simulink model "BRLab"  (R2022b)
settings: Solver=FixedStepDiscrete  StartTime=0.0  StopTime=60  FixedStep=0.01  RelTol=1e-3
undefined symbols (not defined in the file or in its folder): controller, DiscIntNeverNeededParam, drv, filt, gbox, sens, Ts, wheel, yaw
settings Model: Creator=Alessandro  LastModifiedBy=michael
settings SolverCC: AlgebraicLoopSolver=TrustRegion
settings ModelReferenceCC: EnableRefExpFcnMdlSchedulingChecks=on
settings RTWCC: DLArmComputeVersion=19.05

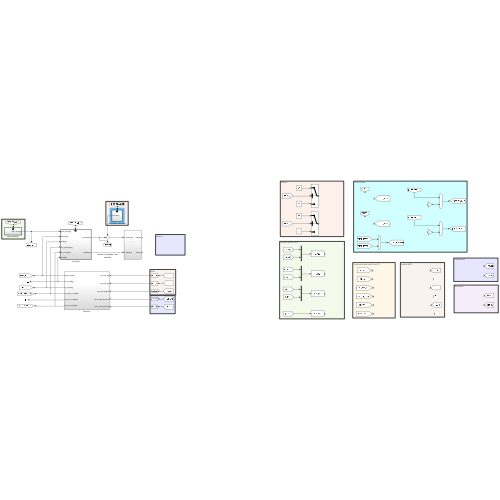
[thumbnail: Simulink's stored preview of the top-level diagram]
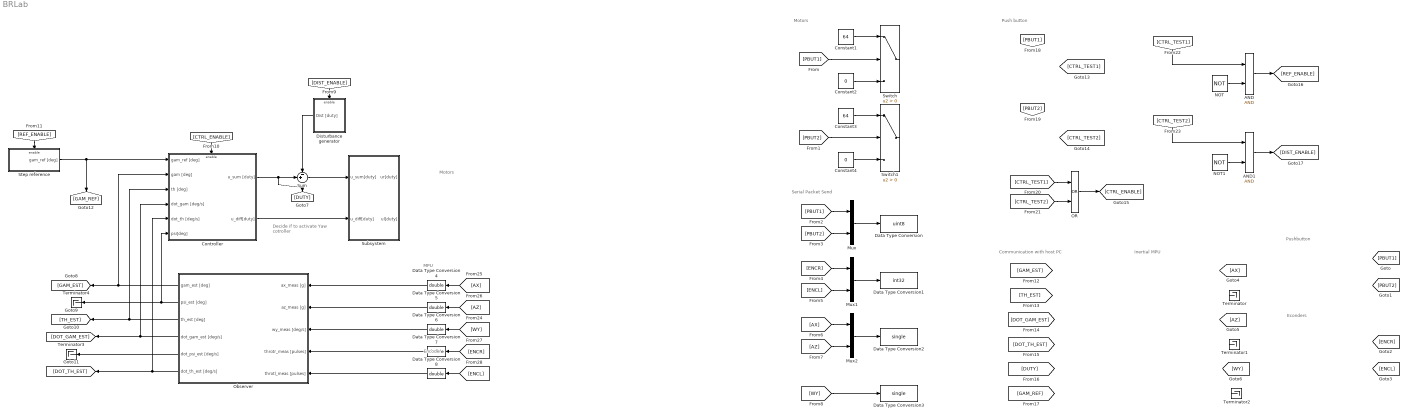
== system BRLab ==
  note: Encoder
  note: MPU
  note: Push button
  note: Communication with host PC
  note: Motors
  note: Decide if to activate Yaw cotroller
  note: Serial Packet Send
  note: Econders
  note: Pushbutton
  note: Motors
  note: Inertial MPU
  AND : Logic  IconShape=distinctive  AllPortsSameDT=off  OutDataTypeStr=boolean
  AND1 : Logic  IconShape=distinctive  AllPortsSameDT=off  OutDataTypeStr=boolean
  Constant1 : Constant  Value=64
  Constant2 : Constant  Value=0
  Constant3 : Constant  Value=64
  Constant4 : Constant  Value=0
  Controller : Subsystem
  Data Type Conversion : DataTypeConversion  OutDataTypeStr=uint8  SaturateOnIntegerOverflow=off  RndMeth=Floor
  Data Type Conversion1 : DataTypeConversion  OutDataTypeStr=int32  SaturateOnIntegerOverflow=off  RndMeth=Floor
  Data Type Conversion2 : DataTypeConversion  OutDataTypeStr=single  SaturateOnIntegerOverflow=off  RndMeth=Floor
  Data Type Conversion3 : DataTypeConversion  OutDataTypeStr=single  SaturateOnIntegerOverflow=off  RndMeth=Floor
  Data Type Conversion{4..8} (5 alike) : DataTypeConversion  OutDataTypeStr=double  SaturateOnIntegerOverflow=off  RndMeth=Floor
  Disturbance generator : Subsystem
  Mux : Mux  Inputs=2
  Mux1 : Mux  Inputs=2
  Mux2 : Mux  Inputs=2
  NOT : Logic  Operator=NOT  IconShape=distinctive  AllPortsSameDT=off  OutDataTypeStr=boolean
  NOT1 : Logic  Operator=NOT  IconShape=distinctive  AllPortsSameDT=off  OutDataTypeStr=boolean
  OR : Logic  Operator=OR  IconShape=distinctive  AllPortsSameDT=off  OutDataTypeStr=boolean
  Observer : Subsystem
  "Step reference " : Subsystem
  Subsystem : Subsystem
  Sum : Sum  Inputs=-+|
  Switch : Switch  Criteria=u2 > Threshold  SaturateOnIntegerOverflow=off  InputSameDT=off
  Switch1 : Switch  Criteria=u2 > Threshold  SaturateOnIntegerOverflow=off  InputSameDT=off
  Terminator{,1..4} (5 alike) : Terminator
  wires:
  Controller/1(u_sum [duty]) -> [DUTY], Sum/2
  Observer/1(gam_est [deg]) -> Controller/2(gam [deg]), [GAM_EST]
  Sum/1 -> Subsystem/1(u_sum[duty])
  Observer/3(th_est [deg]) -> Controller/3(th [deg]), [TH_EST]
  Observer/6(dot_th_est [deg/s]) -> Controller/5(dot_th [deg/s]), [DOT_TH_EST]
  Observer/4(dot_gam_est [deg/s]) -> Controller/4(dot_gam [deg/s]), [DOT_GAM_EST]
  Observer/2(psi_est [deg]) -> Controller/6(psi[deg]), Terminator4/1
  "Step reference "/1(gam_ref [deg]) -> [GAM_REF], Controller/1(gam_ref [deg])
  Controller/2(u_diff[duty]) -> Subsystem/2(u_diff[duty])
  [PBUT1] -> Mux/1
  [WY] -> Data Type Conversion3/1
  Constant1/1 -> Switch/1
  [PBUT1] -> Switch/2
  Constant3/1 -> Switch1/1
  Mux/1 -> Data Type Conversion/1
  [AX] -> Mux2/1
  [ENCL] -> Mux1/2
  [PBUT2] -> Mux/2
  [ENCR] -> Mux1/1
  Mux1/1 -> Data Type Conversion1/1
  Constant4/1 -> Switch1/3
  [PBUT2] -> Switch1/2
  Constant2/1 -> Switch/3
  Mux2/1 -> Data Type Conversion2/1
  [AZ] -> Mux2/2
  Disturbance generator/1(Dist [duty]) -> Sum/1
  [DIST_ENABLE] -> Disturbance generator/Enable
  [CTRL_ENABLE] -> Controller/Enable
  [REF_ENABLE] -> "Step reference "/Enable
  Observer/5(dot_psi_est [deg/s]) -> Terminator3/1
  [CTRL_TEST1] -> OR/1
  [CTRL_TEST2] -> OR/2
  OR/1 -> [CTRL_ENABLE]
  NOT/1 -> AND/2
  [CTRL_TEST1] -> AND/1
  AND/1 -> [REF_ENABLE]
  AND1/1 -> [DIST_ENABLE]
  NOT1/1 -> AND1/2
  [CTRL_TEST2] -> AND1/1
  Data Type Conversion5/1 -> Observer/2(az_meas [g])
  Data Type Conversion4/1 -> Observer/1(ax_meas [g])
  Data Type Conversion6/1 -> Observer/3(wy_meas [deg/s])
  [WY] -> Data Type Conversion6/1
  [AX] -> Data Type Conversion4/1
  [AZ] -> Data Type Conversion5/1
  Data Type Conversion7/1 -> Observer/4(throtr_meas [pulses])
  [ENCR] -> Data Type Conversion7/1
  [ENCL] -> Data Type Conversion8/1
  Data Type Conversion8/1 -> Observer/5(throtl_meas [pulses])

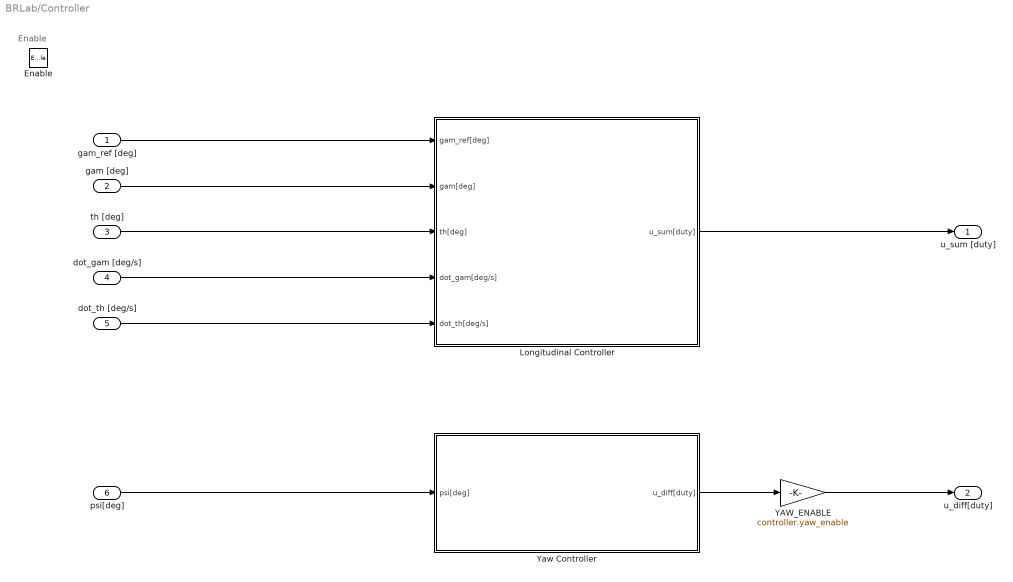
== system BRLab/Controller ==
  note: Enable
  gam_ref [deg] : Inport
  gam [deg] : Inport  Port=2
  th [deg] : Inport  Port=3
  dot_gam [deg/s] : Inport  Port=4
  dot_th [deg/s] : Inport  Port=5
  psi[deg] : Inport  Port=6
  Enable : EnablePort
  Longitudinal Controller : Subsystem
  YAW_ENABLE : Gain  Gain=controller.yaw_enable
  Yaw Controller : Subsystem
  u_sum [duty] : Outport
  u_diff[duty] : Outport  Port=2
  wires:
  psi[deg]/1 -> Yaw Controller/1(psi[deg])
  Yaw Controller/1(u_diff[duty]) -> YAW_ENABLE/1
  gam_ref [deg]/1 -> Longitudinal Controller/1(gam_ref[deg])
  gam [deg]/1 -> Longitudinal Controller/2(gam[deg])
  th [deg]/1 -> Longitudinal Controller/3(th[deg])
  dot_gam [deg/s]/1 -> Longitudinal Controller/4(dot_gam[deg/s])
  dot_th [deg/s]/1 -> Longitudinal Controller/5(dot_th[deg/s])
  Longitudinal Controller/1(u_sum[duty]) -> u_sum [duty]/1
  YAW_ENABLE/1 -> u_diff[duty]/1

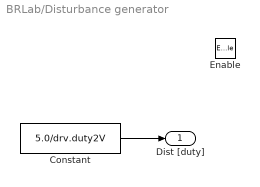
== system BRLab/Disturbance generator ==
  Enable : EnablePort
  Constant : Constant  Value=5.0/drv.duty2V
  Dist [duty] : Outport
  wires:
  Constant/1 -> Dist [duty]/1

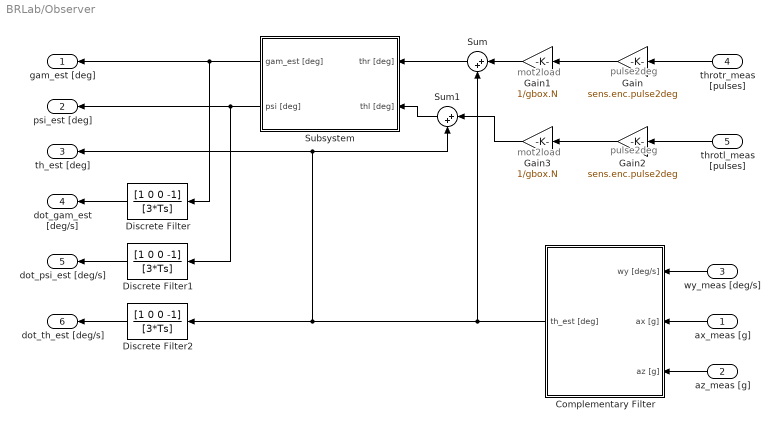
== system BRLab/Observer ==
  note: mot2load
  note: pulse2deg
  note: mot2load
  note: pulse2deg
  ax_meas [g] : Inport
  az_meas [g] : Inport  Port=2
  wy_meas [deg/s] : Inport  Port=3
  throtr_meas [pulses] : Inport  Port=4
  throtl_meas [pulses] : Inport  Port=5
  Complementary Filter : Subsystem
  Discrete Filter : DiscreteFilter  Numerator=[1 0 0 -1]  Denominator=[3*Ts]  SampleTime=Ts
  Discrete Filter1 : DiscreteFilter  Numerator=[1 0 0 -1]  Denominator=[3*Ts]  SampleTime=Ts
  Discrete Filter2 : DiscreteFilter  Numerator=[1 0 0 -1]  Denominator=[3*Ts]  SampleTime=Ts
  Gain : Gain  Gain=sens.enc.pulse2deg
  Gain1 : Gain  Gain=1/gbox.N
  Gain2 : Gain  Gain=sens.enc.pulse2deg
  Gain3 : Gain  Gain=1/gbox.N
  Subsystem : Subsystem
  Sum : Sum  Inputs=|++
  Sum1 : Sum  Inputs=|++
  gam_est [deg] : Outport
  psi_est [deg] : Outport  Port=2
  th_est [deg] : Outport  Port=3
  dot_gam_est [deg/s] : Outport  Port=4
  dot_psi_est [deg/s] : Outport  Port=5
  dot_th_est [deg/s] : Outport  Port=6
  wires:
  Discrete Filter/1 -> dot_gam_est [deg/s]/1
  Gain1/1 -> Sum/1
  Discrete Filter1/1 -> dot_psi_est [deg/s]/1
  Gain/1 -> Gain1/1
  throtr_meas [pulses]/1 -> Gain/1
  wy_meas [deg/s]/1 -> Complementary Filter/1(wy [deg/s])
  Gain2/1 -> Gain3/1
  throtl_meas [pulses]/1 -> Gain2/1
  Gain3/1 -> Sum1/1
  Sum/1 -> Subsystem/1(thr [deg])
  Sum1/1 -> Subsystem/2(thl [deg])
  Complementary Filter/1(th_est [deg]) -> Sum1/2, th_est [deg]/1, Discrete Filter2/1, Sum/2
  Subsystem/2(psi [deg]) -> Discrete Filter1/1, psi_est [deg]/1
  Subsystem/1(gam_est [deg]) -> Discrete Filter/1, gam_est [deg]/1
  Discrete Filter2/1 -> dot_th_est [deg/s]/1
  ax_meas [g]/1 -> Complementary Filter/2(ax [g])
  az_meas [g]/1 -> Complementary Filter/3(az [g])

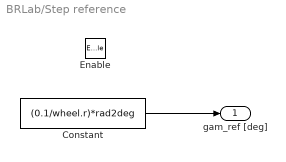
== system BRLab/Step reference  ==
  Enable : EnablePort
  Constant : Constant  Value=(0.1/wheel.r)*rad2deg
  gam_ref [deg] : Outport
  wires:
  Constant/1 -> gam_ref [deg]/1

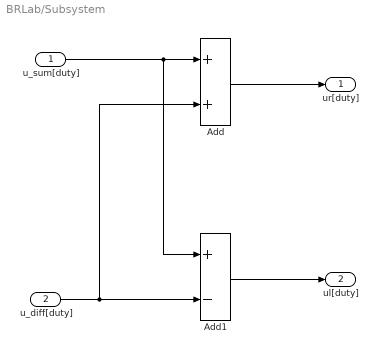
== system BRLab/Subsystem ==
  u_sum[duty] : Inport
  u_diff[duty] : Inport  Port=2
  Add : Sum
  Add1 : Sum  Inputs=+-
  ur[duty] : Outport
  ul[duty] : Outport  Port=2
  wires:
  u_diff[duty]/1 -> Add/2, Add1/2
  Add/1 -> ur[duty]/1
  u_sum[duty]/1 -> Add1/1, Add/1
  Add1/1 -> ul[duty]/1

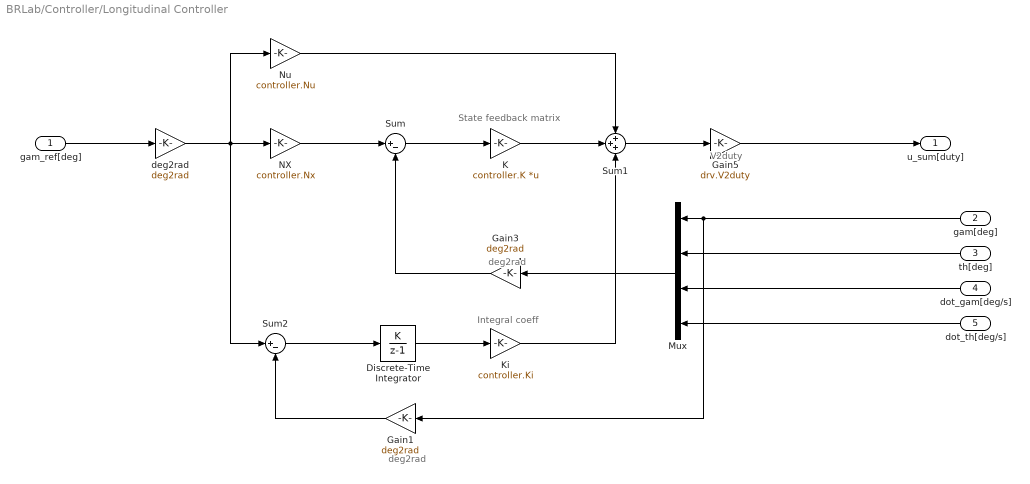
== system BRLab/Controller/Longitudinal Controller ==
  note: State feedback matrix
  note: Integral coeff
  note: V2duty
  note: deg2rad
  note: deg2rad
  gam_ref[deg] : Inport
  gam[deg] : Inport  Port=2
  th[deg] : Inport  Port=3
  dot_gam[deg/s] : Inport  Port=4
  dot_th[deg/s] : Inport  Port=5
  Discrete-Time Integrator : DiscreteIntegrator  IntegratorMethod=Accumulation: Forward Euler  SampleTime=-1  ICPrevOutput=DiscIntNeverNeededParam  ICPrevScaledInput=DiscIntNeverNeededParam
  Gain1 : Gain  Gain=deg2rad
  Gain3 : Gain  Gain=deg2rad
  Gain5 : Gain  Gain=drv.V2duty
  K : Gain  Gain=controller.K  Multiplication=Matrix(K*u)
  Ki : Gain  Gain=controller.Ki
  Mux : Mux
  NX : Gain  Gain=controller.Nx
  Nu : Gain  Gain=controller.Nu
  Sum : Sum  Inputs=|+-
  Sum1 : Sum  Inputs=+++
  Sum2 : Sum  Inputs=|+-
  deg2rad : Gain  Gain=deg2rad
  u_sum[duty] : Outport
  wires:
  Discrete-Time Integrator/1 -> Ki/1
  dot_gam[deg/s]/1 -> Mux/3
  Sum2/1 -> Discrete-Time Integrator/1
  dot_th[deg/s]/1 -> Mux/4
  th[deg]/1 -> Mux/2
  gam_ref[deg]/1 -> deg2rad/1
  Ki/1 -> Sum1/3
  Nu/1 -> Sum1/1
  Gain5/1 -> u_sum[duty]/1
  Gain1/1 -> Sum2/2
  Mux/1 -> Gain3/1
  NX/1 -> Sum/1
  Sum1/1 -> Gain5/1
  Sum/1 -> K/1
  K/1 -> Sum1/2
  Gain3/1 -> Sum/2
  gam[deg]/1 -> Gain1/1, Mux/1
  deg2rad/1 -> NX/1, Nu/1, Sum2/1

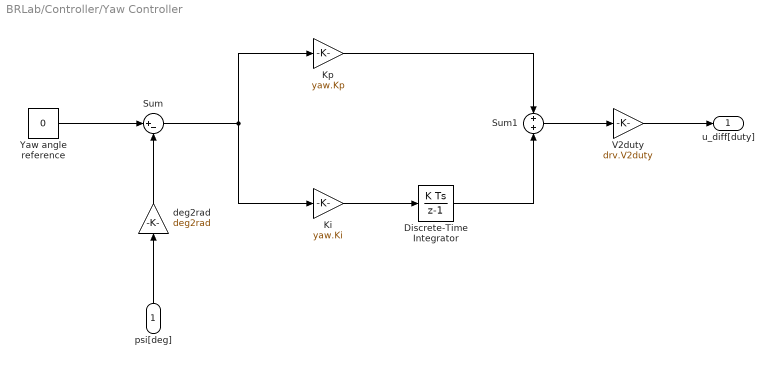
== system BRLab/Controller/Yaw Controller ==
  psi[deg] : Inport
  Discrete-Time Integrator : DiscreteIntegrator  SampleTime=Ts  ICPrevOutput=DiscIntNeverNeededParam  ICPrevScaledInput=DiscIntNeverNeededParam
  Ki : Gain  Gain=yaw.Ki
  Kp : Gain  Gain=yaw.Kp
  Sum : Sum  Inputs=|+-
  Sum1 : Sum  Inputs=+|+
  V2duty : Gain  Gain=drv.V2duty
  Yaw angle reference : Constant  Value=0
  deg2rad : Gain  Gain=deg2rad
  u_diff[duty] : Outport
  wires:
  deg2rad/1 -> Sum/2
  psi[deg]/1 -> deg2rad/1
  Yaw angle reference/1 -> Sum/1
  Sum/1 -> Kp/1, Ki/1
  Sum1/1 -> V2duty/1
  V2duty/1 -> u_diff[duty]/1
  Kp/1 -> Sum1/1
  Discrete-Time Integrator/1 -> Sum1/2
  Ki/1 -> Discrete-Time Integrator/1

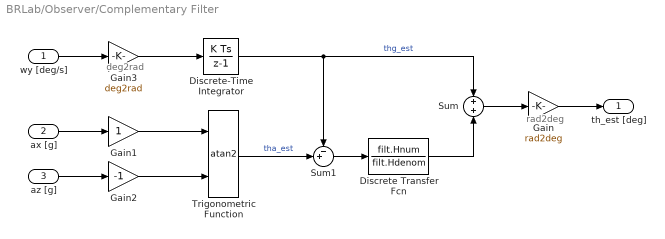
== system BRLab/Observer/Complementary Filter ==
  note: rad2deg
  note: deg2rad
  wy [deg/s] : Inport
  ax [g] : Inport  Port=2
  az [g] : Inport  Port=3
  Discrete Transfer Fcn : DiscreteTransferFcn  Numerator=filt.Hnum  Denominator=filt.Hdenom  SampleTime=Ts
  Discrete-Time Integrator : DiscreteIntegrator  SampleTime=Ts  ICPrevOutput=DiscIntNeverNeededParam  ICPrevScaledInput=DiscIntNeverNeededParam
  Gain : Gain  Gain=rad2deg
  Gain1 : Gain
  Gain2 : Gain  Gain=-1
  Gain3 : Gain  Gain=deg2rad
  Sum : Sum  Inputs=+|+
  Sum1 : Sum  Inputs=-+|
  Trigonometric Function : Trigonometry  Operator=atan2
  th_est [deg] : Outport
  wires:
  Gain/1 -> th_est [deg]/1
  Sum/1 -> Gain/1
  ax [g]/1 -> Gain1/1
  Gain1/1 -> Trigonometric Function/1
  az [g]/1 -> Gain2/1
  Gain2/1 -> Trigonometric Function/2
  wy [deg/s]/1 -> Gain3/1
  Gain3/1 -> Discrete-Time Integrator/1
  Trigonometric Function/1 -> Sum1/2  "tha_est"
  Discrete-Time Integrator/1 -> Sum/1, Sum1/1  "thg_est"
  Sum1/1 -> Discrete Transfer Fcn/1
  Discrete Transfer Fcn/1 -> Sum/2

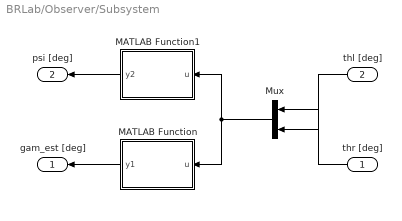
== system BRLab/Observer/Subsystem ==
  thr [deg] : Inport
  thl [deg] : Inport  Port=2
  MATLAB Function : MATLAB Function  TreatAsAtomicUnit=on
  MATLAB Function1 : MATLAB Function  TreatAsAtomicUnit=on
  Mux : Mux  Inputs=2
  gam_est [deg] : Outport
  psi [deg] : Outport  Port=2
  wires:
  MATLAB Function1/1(y2) -> psi [deg]/1
  MATLAB Function/1(y1) -> gam_est [deg]/1
  Mux/1 -> MATLAB Function/1(u), MATLAB Function1/1(u)
  thr [deg]/1 -> Mux/1
  thl [deg]/1 -> Mux/2

== matlab function BRLab/Observer/Subsystem/MATLAB Function ==
  data: u input; y1 output
function y1 = gam_angle(u)

y1=(u(1)+u(2))/2;

== matlab function BRLab/Observer/Subsystem/MATLAB Function1 ==
  data: u input; y2 output
function y2 = psi_angle(u)
wheel.r = 0.034;
wheel.yb=0.1;
w=2*abs(wheel.yb);

y2 = (wheel.r/w)*(u(1)-u(2));
